simulink model "ZT_VehCtrl_18B"  (R2018b)
settings: Solver=FixedStepAuto  StartTime=0.0  StopTime=inf  FixedStep=0.005  RelTol=1e-3
InitFcn:
  | mbd_mpc_consistency_checks(bdroot(gcs));
undefined symbols (not defined in the file or in its folder): ANG_DEAD, BMS_NormalPwr, BrkPrsByBrkPct_TB_X, BrkPrsByBrkPct_TB_Y, DELAY_DISCHARGE, DELAY_RCUOFF, DRV_BACKWARD, DRV_BRAKE, DRV_FORWARD, DRV_NEUTRAL, DRV_PARK, DRV_UNPARK, DRV_ZEROTURN, EPB_LOCK, EPB_UNLOCK, ExtraLoadPwr, FanOff, fifo_0_vect, fifo_1_vect, HiFanReq, HV_finished, HV_No_Active, HV_POWER_OFF, HV_POWER_ON, HVDown, HVON, KaTLS_v_DrgUp_X_VehSpd, KeFTM_s_Way1OffDlyTime, KeFTM_TK_Way1CoolLv2OffBatTemp, KeFTM_TK_Way1CoolLv2OffMtrTemp, KeFTM_TK_Way1CoolLv2OnBatTemp, KeFTM_TK_Way1CoolLv2OnMtrTemp, KeFTM_TK_Way1CoolLv3OffBatTemp, KeFTM_TK_Way1CoolLv3OffMtrTemp, KeFTM_TK_Way1CoolLv3OnBatTemp, KeFTM_TK_Way1CoolLv3OnMtrTemp, KeFTM_TK_Way1CoolLv4OffBatTemp, KeFTM_TK_Way1CoolLv4OffMtrTemp, KeFTM_TK_Way1CoolLv4OnBatTemp, KeFTM_TK_Way1CoolLv4OnMtrTemp, Kp1, Kp2, LowFanReq, LQFP, MtrPwrFactor_RCU, MtrPwrHighToMidThd, MtrPwrLowToMidThd, MtrPwrMidToHighThd, MtrPwrMidToLowThd, MtrTrqMax, PCT_DEAD, Precharge, PTO_1000, PTO_540, pts1_fifo_0_vect, pts1_fifo_1_vect, pts2_fifo_0_vect, pts2_fifo_1_vect, pts3_fifo_0_vect, pts3_fifo_1_vect ... (+24)
libraries: mbd_mpc574x_ec_toolbox x173, canmsglib x72, simulink x57
(part 3 of 12)

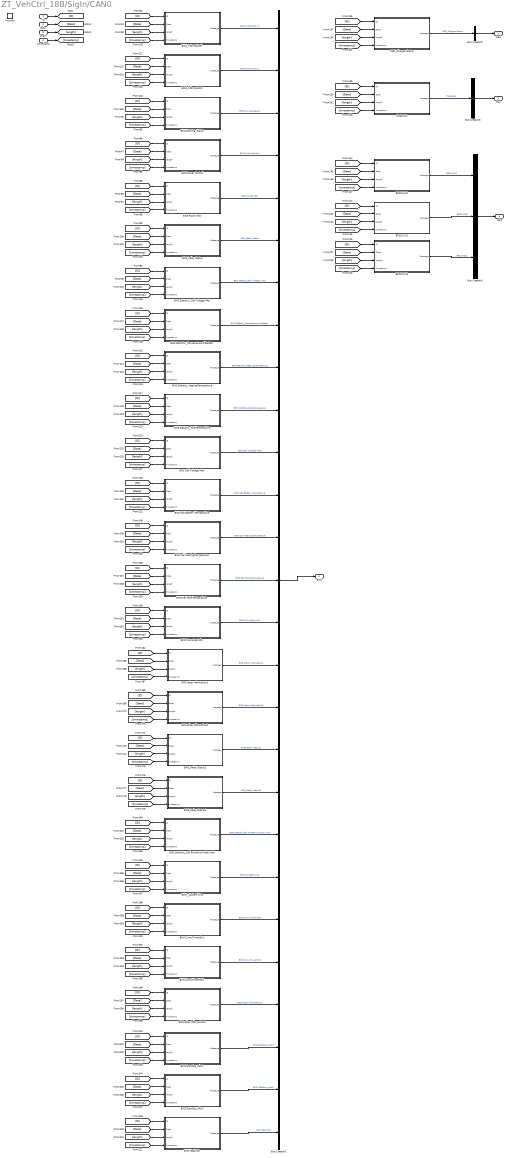
== system ZT_VehCtrl_18B/SigIn/CAN0  ==
  ID : Inport
  Data : Inport  Port=2
  length : Inport  Port=3
  timestamp : Inport  Port=4
  function : TriggerPort  TriggerType=function-call  VariantControl=Variant
  BMS Cell Battery Temperature : Subsystem
  BMS Cell HeatingTemperature : Subsystem
  BMS Cell Pole Temperature : Subsystem
  BMS Cell Voltage Infor : Subsystem
  BMS CumuCap Infor : Subsystem
  BMS CumuTimeInfor1 : Subsystem
  BMS CumuTimeInfor2 : Subsystem
  BMS HeatInfor : Subsystem
  BMS Power Control : Subsystem
  BMS Power Infor : Subsystem
  BMS StartDia_Infor1 : Subsystem
  BMS StartDia_Infor2 : Subsystem
  BMS Statistic_Cell ExtremumIndex Infor : Subsystem
  BMS Statistic_Cell Voltage Infor : Subsystem
  BMS Statistic_HeatingTemperature : Subsystem
  BMS Statistic_PoleTemperature : Subsystem
  BMS Statistic_Temperature of Battery : Subsystem
  "BMS _SystemTime " : Subsystem
  BMS other Information1 : Subsystem
  "BMS other Information2 " : Subsystem
  BMS other Information3 : Subsystem
  BMSWarning_Status : Subsystem
  BMS_Information1 : Subsystem
  BMS_Information2 : Subsystem
  BMS_Relay Status : Subsystem
  BMS_Relay Status2 : Subsystem
  BMS_Relay Status3 : Subsystem
  BRS2VCU1 : Subsystem
  BRS2VCU2 : Subsystem
  BRS2VCU3 : Subsystem
  Bus Creator5 : BusCreator  Inputs=27
  Bus Creator6 : BusCreator  Inputs=1
  Bus Creator8 : BusCreator  Inputs=1
  Bus Creator9 : BusCreator  Inputs=3
  OBC_Charger Status : Subsystem
  TMS2VCU : Subsystem
  BMS : Outport
  OBC : Outport  Port=2
  TMS : Outport  Port=3
  "BRS " : Outport  Port=4
  wires:
  [timestamp] -> BMS Statistic_Temperature of Battery/4(timestamp)
  [ID] -> BMS Cell Battery Temperature/1(ID)
  BMS Statistic_PoleTemperature/1(Message) -> Bus Creator5/10  "BMS Statistic_PoleTemperature"
  [Data] -> BMS_Relay Status/2(Data)
  BMS Statistic_Temperature of Battery/1(Message) -> Bus Creator5/8  "BMS Statistic_Temperature of Battery"
  BMS Statistic_HeatingTemperature/1(Message) -> Bus Creator5/9  "BMS Statistic_HeatingTemperature"
  [length] -> BMS Cell Battery Temperature/3(length)
  [timestamp] -> BMS Statistic_Cell Voltage Infor/4(timestamp)
  [length] -> BMS Statistic_Temperature of Battery/3(length)
  BMS Power Infor/1(Message) -> Bus Creator5/5  "BMS Power Infor"
  [timestamp] -> BMS Cell Battery Temperature/4(timestamp)
  [ID] -> BMS Statistic_PoleTemperature/1(ID)
  BMS Cell Battery Temperature/1(Message) -> Bus Creator5/12  "BMS Cell Battery Temperature"
  [Data] -> BMS Statistic_Cell Voltage Infor/2(Data)
  [length] -> BMS Statistic_PoleTemperature/3(length)
  [timestamp] -> BMS Statistic_PoleTemperature/4(timestamp)
  [Data] -> BMS Power Control/2(Data)
  [Data] -> BMS Statistic_PoleTemperature/2(Data)
  [Data] -> BMS Cell Voltage Infor/2(Data)
  BMS_Relay Status/1(Message) -> Bus Creator5/6  "BMS_Relay Status"
  [timestamp] -> BMSWarning_Status/4(timestamp)
  [ID] -> BMS Statistic_Cell Voltage Infor/1(ID)
  [Data] -> BMS Statistic_Temperature of Battery/2(Data)
  [length] -> BMSWarning_Status/3(length)
  [timestamp] -> BMS Statistic_HeatingTemperature/4(timestamp)
  Bus Creator5/1 -> BMS/1
  [timestamp] -> BMS Power Control/4(timestamp)
  [Data] -> BMS Statistic_HeatingTemperature/2(Data)
  [ID] -> BMS Power Control/1(ID)
  [Data] -> BMS Power Infor/2(Data)
  BMS Statistic_Cell Voltage Infor/1(Message) -> Bus Creator5/7  "BMS Statistic_Cell Voltage Infor"
  [ID] -> BMSWarning_Status/1(ID)
  [Data] -> BMS Cell Battery Temperature/2(Data)
  [Data] -> BMSWarning_Status/2(Data)
  [length] -> BMS Power Control/3(length)
  [ID] -> BMS Cell Voltage Infor/1(ID)
  BMSWarning_Status/1(Message) -> Bus Creator5/3  "BMSWarning_Status"
  [timestamp] -> BMS Cell Voltage Infor/4(timestamp)
  [length] -> BMS Statistic_HeatingTemperature/3(length)
  [timestamp] -> BMS_Relay Status/4(timestamp)
  [ID] -> BMS Statistic_HeatingTemperature/1(ID)
  [length] -> BMS Statistic_Cell Voltage Infor/3(length)
  [length] -> BMS_Relay Status/3(length)
  BMS Power Control/1(Message) -> Bus Creator5/4  "BMS Power Control"
  [ID] -> BMS Power Infor/1(ID)
  [length] -> BMS Cell Voltage Infor/3(length)
  [timestamp] -> BMS Power Infor/4(timestamp)
  [ID] -> BMS Statistic_Temperature of Battery/1(ID)
  BMS Cell Voltage Infor/1(Message) -> Bus Creator5/11  "BMS Cell Voltage Infor"
  [ID] -> BMS_Relay Status/1(ID)
  [length] -> BMS Power Infor/3(length)
  [Data] -> OBC_Charger Status/2(Data)
  OBC_Charger Status/1(Message) -> Bus Creator6/1  "OBC_Charger Status"
  [length] -> OBC_Charger Status/3(length)
  [ID] -> OBC_Charger Status/1(ID)
  Bus Creator6/1 -> OBC/1
  [timestamp] -> OBC_Charger Status/4(timestamp)
  BMS_Information2/1(Message) -> Bus Creator5/2  "BMS_Information2"
  BMS_Information1/1(Message) -> Bus Creator5/1  "BMS_Information1"
  [ID] -> BMS_Information2/1(ID)
  [Data] -> BMS_Information2/2(Data)
  [length] -> BMS_Information2/3(length)
  [timestamp] -> BMS_Information1/4(timestamp)
  [length] -> BMS_Information1/3(length)
  [Data] -> BMS_Information1/2(Data)
  [ID] -> BMS_Information1/1(ID)
  [timestamp] -> BMS_Information2/4(timestamp)
  [Data] -> BMS Cell HeatingTemperature/2(Data)
  BMS Cell HeatingTemperature/1(Message) -> Bus Creator5/13  "BMS Cell HeatingTemperature"
  [timestamp] -> BMS Cell HeatingTemperature/4(timestamp)
  [length] -> BMS Cell HeatingTemperature/3(length)
  [ID] -> BMS Cell HeatingTemperature/1(ID)
  [ID] -> BMS Cell Pole Temperature/1(ID)
  [length] -> BMS Cell Pole Temperature/3(length)
  [timestamp] -> BMS Cell Pole Temperature/4(timestamp)
  BMS Cell Pole Temperature/1(Message) -> Bus Creator5/14  "BMS Cell Pole Temperature"
  [Data] -> BMS Cell Pole Temperature/2(Data)
  [Data] -> BMS CumuCap Infor/2(Data)
  BMS CumuCap Infor/1(Message) -> Bus Creator5/15  "BMS CumuCap Infor"
  [timestamp] -> BMS CumuCap Infor/4(timestamp)
  [length] -> BMS CumuCap Infor/3(length)
  [ID] -> BMS CumuCap Infor/1(ID)
  [ID] -> BMS other Information1/1(ID)
  [length] -> BMS other Information1/3(length)
  [timestamp] -> BMS other Information1/4(timestamp)
  BMS other Information1/1(Message) -> Bus Creator5/16  "BMS other Information1"
  [Data] -> BMS other Information1/2(Data)
  [Data] -> "BMS other Information2 "/2(Data)
  "BMS other Information2 "/1(Message) -> Bus Creator5/17  "BMS other Information2"
  [timestamp] -> "BMS other Information2 "/4(timestamp)
  [length] -> "BMS other Information2 "/3(length)
  [ID] -> "BMS other Information2 "/1(ID)
  [ID] -> BMS_Relay Status2/1(ID)
  [length] -> BMS_Relay Status2/3(length)
  [timestamp] -> BMS_Relay Status2/4(timestamp)
  BMS_Relay Status2/1(Message) -> Bus Creator5/18  "BMS_Relay Status2"
  [Data] -> BMS_Relay Status2/2(Data)
  [Data] -> BMS_Relay Status3/2(Data)
  BMS_Relay Status3/1(Message) -> Bus Creator5/19  "BMS_Relay Status3"
  [timestamp] -> BMS_Relay Status3/4(timestamp)
  [length] -> BMS_Relay Status3/3(length)
  [ID] -> BMS_Relay Status3/1(ID)
  [ID] -> BMS Statistic_Cell ExtremumIndex Infor/1(ID)
  [length] -> BMS Statistic_Cell ExtremumIndex Infor/3(length)
  [timestamp] -> BMS Statistic_Cell ExtremumIndex Infor/4(timestamp)
  BMS Statistic_Cell ExtremumIndex Infor/1(Message) -> Bus Creator5/20  "BMS Statistic_Cell ExtremumIndex Infor"
  [Data] -> BMS Statistic_Cell ExtremumIndex Infor/2(Data)
  [Data] -> "BMS _SystemTime "/2(Data)
  "BMS _SystemTime "/1(Message) -> Bus Creator5/21  "BMS _SystemTime"
  [timestamp] -> "BMS _SystemTime "/4(timestamp)
  [length] -> "BMS _SystemTime "/3(length)
  [ID] -> "BMS _SystemTime "/1(ID)
  [ID] -> BMS CumuTimeInfor1/1(ID)
  [length] -> BMS CumuTimeInfor1/3(length)
  [timestamp] -> BMS CumuTimeInfor1/4(timestamp)
  BMS CumuTimeInfor1/1(Message) -> Bus Creator5/22  "BMS CumuTimeInfor1"
  [Data] -> BMS CumuTimeInfor1/2(Data)
  [Data] -> BMS CumuTimeInfor2/2(Data)
  BMS CumuTimeInfor2/1(Message) -> Bus Creator5/23  "BMS CumuTimeInfor2"
  [timestamp] -> BMS CumuTimeInfor2/4(timestamp)
  [length] -> BMS CumuTimeInfor2/3(length)
  [ID] -> BMS CumuTimeInfor2/1(ID)
  [ID] -> BMS other Information3/1(ID)
  [length] -> BMS other Information3/3(length)
  [timestamp] -> BMS other Information3/4(timestamp)
  BMS other Information3/1(Message) -> Bus Creator5/24  "BMS other Information3"
  [Data] -> BMS other Information3/2(Data)
  [Data] -> BMS StartDia_Infor1/2(Data)
  BMS StartDia_Infor1/1(Message) -> Bus Creator5/25  "BMS StartDia_Infor1"
  [timestamp] -> BMS StartDia_Infor1/4(timestamp)
  [length] -> BMS StartDia_Infor1/3(length)
  [ID] -> BMS StartDia_Infor1/1(ID)
  [ID] -> BMS StartDia_Infor2/1(ID)
  [length] -> BMS StartDia_Infor2/3(length)
  [timestamp] -> BMS StartDia_Infor2/4(timestamp)
  BMS StartDia_Infor2/1(Message) -> Bus Creator5/26  "BMS StartDia_Infor2"
  [Data] -> BMS StartDia_Infor2/2(Data)
  [Data] -> BMS HeatInfor/2(Data)
  BMS HeatInfor/1(Message) -> Bus Creator5/27  "BMS HeatInfor"
  [timestamp] -> BMS HeatInfor/4(timestamp)
  [length] -> BMS HeatInfor/3(length)
  [ID] -> BMS HeatInfor/1(ID)
  [timestamp] -> TMS2VCU/4(timestamp)
  Bus Creator8/1 -> TMS/1
  [ID] -> TMS2VCU/1(ID)
  [length] -> TMS2VCU/3(length)
  TMS2VCU/1(Message) -> Bus Creator8/1  "TMS2VCU"
  [Data] -> TMS2VCU/2(Data)
  [Data] -> BRS2VCU1/2(Data)
  BRS2VCU1/1(Message) -> Bus Creator9/1  "BRS2VCU1"
  [length] -> BRS2VCU1/3(length)
  [ID] -> BRS2VCU1/1(ID)
  Bus Creator9/1 -> "BRS "/1
  [timestamp] -> BRS2VCU1/4(timestamp)
  [timestamp] -> BRS2VCU2/4(timestamp)
  [ID] -> BRS2VCU2/1(ID)
  [length] -> BRS2VCU2/3(length)
  [Data] -> BRS2VCU2/2(Data)
  [Data] -> BRS2VCU3/2(Data)
  [length] -> BRS2VCU3/3(length)
  [ID] -> BRS2VCU3/1(ID)
  [timestamp] -> BRS2VCU3/4(timestamp)
  BRS2VCU2/1(Message) -> Bus Creator9/2  "BRS2VCU2"
  BRS2VCU3/1(Message) -> Bus Creator9/3  "BRS2VCU3"
  length/1 -> [length]
  ID/1 -> [ID]
  timestamp/1 -> [timestamp]
  Data/1 -> [Data]

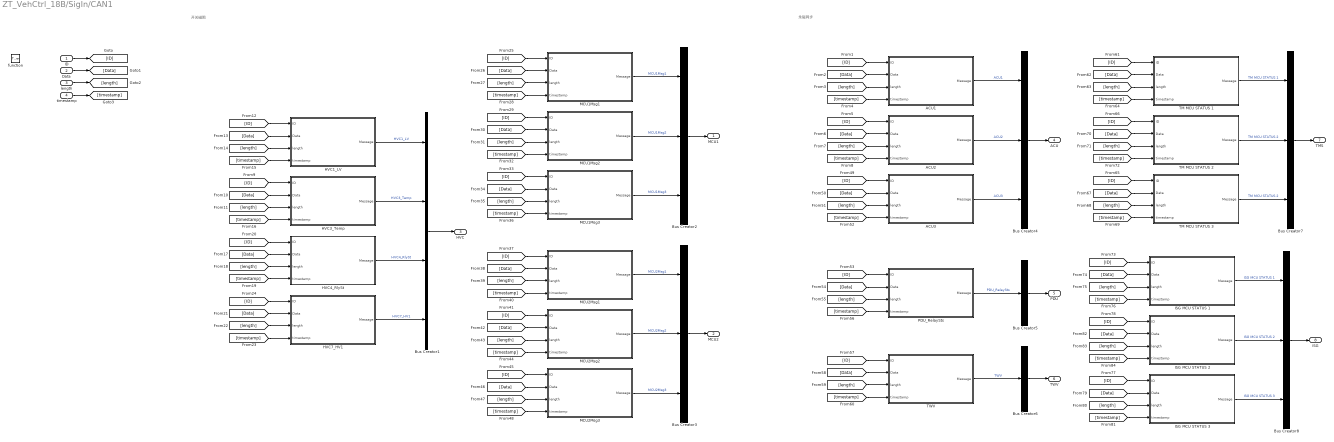
== system ZT_VehCtrl_18B/SigIn/CAN1 ==
  note: 永磁同步
  note: 开关磁阻
  ID : Inport
  Data : Inport  Port=2
  length : Inport  Port=3
  timestamp : Inport  Port=4
  function : TriggerPort  TriggerType=function-call  VariantControl=Variant
  ACU1 : Subsystem
  ACU2 : Subsystem
  ACU3 : Subsystem
  Bus Creator1 : BusCreator  Inputs=4
  Bus Creator{2..4,7..8} (5 alike) : BusCreator  Inputs=3
  Bus Creator5 : BusCreator  Inputs=1
  Bus Creator6 : BusCreator  Inputs=1
  HVC1_LV : Subsystem
  HVC3_Temp : Subsystem
  HVC4_RlySt : Subsystem
  HVC7_HV1 : Subsystem
  ISG MCU STATUS 1 : Subsystem
  ISG MCU STATUS 2 : Subsystem
  ISG MCU STATUS 3 : Subsystem
  MCU1Msg1 : Subsystem
  MCU1Msg2 : Subsystem
  MCU1Msg3 : Subsystem
  MCU2Msg1 : Subsystem
  MCU2Msg2 : Subsystem
  MCU2Msg3 : Subsystem
  PDU_RelaySts : Subsystem
  TM MCU STATUS 1 : Subsystem
  TM MCU STATUS 2 : Subsystem
  TM MCU STATUS 3 : Subsystem
  "TWV " : Subsystem
  MCU1 : Outport
  MCU2 : Outport  Port=2
  HVC : Outport  Port=3
  ACU : Outport  Port=4
  PDU : Outport  Port=5
  TWV : Outport  Port=6
  TMS : Outport  Port=7
  "ISG " : Outport  Port=8
  wires:
  length/1 -> [length]
  timestamp/1 -> [timestamp]
  Data/1 -> [Data]
  ID/1 -> [ID]
  Bus Creator2/1 -> MCU1/1
  [Data] -> HVC1_LV/2(Data)
  [timestamp] -> HVC1_LV/4(timestamp)
  [ID] -> HVC1_LV/1(ID)
  HVC1_LV/1(Message) -> Bus Creator1/1  "HVC1_LV"
  [length] -> HVC1_LV/3(length)
  [length] -> HVC3_Temp/3(length)
  HVC3_Temp/1(Message) -> Bus Creator1/2  "HVC3_Temp"
  [ID] -> HVC3_Temp/1(ID)
  [timestamp] -> HVC3_Temp/4(timestamp)
  [Data] -> HVC3_Temp/2(Data)
  [Data] -> HVC4_RlySt/2(Data)
  [timestamp] -> HVC4_RlySt/4(timestamp)
  [ID] -> HVC4_RlySt/1(ID)
  [length] -> HVC4_RlySt/3(length)
  HVC4_RlySt/1(Message) -> Bus Creator1/3  "HVC4_RlySt"
  HVC7_HV1/1(Message) -> Bus Creator1/4  "HVC7_HV1"
  [length] -> HVC7_HV1/3(length)
  [ID] -> HVC7_HV1/1(ID)
  [timestamp] -> HVC7_HV1/4(timestamp)
  [Data] -> HVC7_HV1/2(Data)
  [length] -> MCU1Msg1/3(length)
  MCU1Msg1/1(Message) -> Bus Creator2/1  "MCU1Msg1"
  [ID] -> MCU1Msg1/1(ID)
  [timestamp] -> MCU1Msg1/4(timestamp)
  [Data] -> MCU1Msg1/2(Data)
  [Data] -> MCU1Msg2/2(Data)
  [timestamp] -> MCU1Msg2/4(timestamp)
  [ID] -> MCU1Msg2/1(ID)
  MCU1Msg2/1(Message) -> Bus Creator2/2  "MCU1Msg2"
  [length] -> MCU1Msg2/3(length)
  [length] -> MCU1Msg3/3(length)
  [ID] -> MCU1Msg3/1(ID)
  [timestamp] -> MCU1Msg3/4(timestamp)
  [Data] -> MCU1Msg3/2(Data)
  MCU1Msg3/1(Message) -> Bus Creator2/3  "MCU1Msg3"
  MCU2Msg3/1(Message) -> Bus Creator3/3  "MCU2Msg3"
  [Data] -> MCU2Msg3/2(Data)
  [timestamp] -> MCU2Msg3/4(timestamp)
  [ID] -> MCU2Msg3/1(ID)
  [length] -> MCU2Msg3/3(length)
  [length] -> MCU2Msg2/3(length)
  MCU2Msg2/1(Message) -> Bus Creator3/2  "MCU2Msg2"
  [ID] -> MCU2Msg2/1(ID)
  [timestamp] -> MCU2Msg2/4(timestamp)
  [Data] -> MCU2Msg2/2(Data)
  [Data] -> MCU2Msg1/2(Data)
  [timestamp] -> MCU2Msg1/4(timestamp)
  [ID] -> MCU2Msg1/1(ID)
  MCU2Msg1/1(Message) -> Bus Creator3/1  "MCU2Msg1"
  [length] -> MCU2Msg1/3(length)
  ACU3/1(Message) -> Bus Creator4/3  "ACU3"
  [Data] -> ACU3/2(Data)
  [timestamp] -> ACU3/4(timestamp)
  [ID] -> ACU3/1(ID)
  [length] -> ACU3/3(length)
  [length] -> ACU2/3(length)
  ACU2/1(Message) -> Bus Creator4/2  "ACU2"
  [ID] -> ACU2/1(ID)
  [timestamp] -> ACU2/4(timestamp)
  [Data] -> ACU2/2(Data)
  [Data] -> ACU1/2(Data)
  [timestamp] -> ACU1/4(timestamp)
  [ID] -> ACU1/1(ID)
  ACU1/1(Message) -> Bus Creator4/1  "ACU1"
  [length] -> ACU1/3(length)
  Bus Creator4/1 -> ACU/1
  [length] -> PDU_RelaySts/3(length)
  [ID] -> PDU_RelaySts/1(ID)
  [timestamp] -> PDU_RelaySts/4(timestamp)
  [Data] -> PDU_RelaySts/2(Data)
  PDU_RelaySts/1(Message) -> Bus Creator5/1  "PDU_RelaySts"
  Bus Creator5/1 -> PDU/1
  Bus Creator6/1 -> TWV/1
  "TWV "/1(Message) -> Bus Creator6/1  "TWV"
  [Data] -> "TWV "/2(Data)
  [timestamp] -> "TWV "/4(timestamp)
  [ID] -> "TWV "/1(ID)
  [length] -> "TWV "/3(length)
  Bus Creator7/1 -> TMS/1
  [length] -> TM MCU STATUS 1/3(length)
  TM MCU STATUS 1/1(Message) -> Bus Creator7/1  "TM MCU STATUS 1"
  [ID] -> TM MCU STATUS 1/1(ID)
  [timestamp] -> TM MCU STATUS 1/4(timestamp)
  [Data] -> TM MCU STATUS 1/2(Data)
  [Data] -> TM MCU STATUS 2/2(Data)
  [timestamp] -> TM MCU STATUS 2/4(timestamp)
  [ID] -> TM MCU STATUS 2/1(ID)
  TM MCU STATUS 2/1(Message) -> Bus Creator7/2  "TM MCU STATUS 2"
  [length] -> TM MCU STATUS 2/3(length)
  [length] -> TM MCU STATUS 3/3(length)
  [ID] -> TM MCU STATUS 3/1(ID)
  [timestamp] -> TM MCU STATUS 3/4(timestamp)
  [Data] -> TM MCU STATUS 3/2(Data)
  TM MCU STATUS 3/1(Message) -> Bus Creator7/3  "TM MCU STATUS 2"
  ISG MCU STATUS 3/1(Message) -> Bus Creator8/3  "ISG MCU STATUS 3"
  [Data] -> ISG MCU STATUS 3/2(Data)
  [timestamp] -> ISG MCU STATUS 3/4(timestamp)
  [ID] -> ISG MCU STATUS 3/1(ID)
  [length] -> ISG MCU STATUS 3/3(length)
  [length] -> ISG MCU STATUS 2/3(length)
  ISG MCU STATUS 2/1(Message) -> Bus Creator8/2  "ISG MCU STATUS 2"
  [ID] -> ISG MCU STATUS 2/1(ID)
  [timestamp] -> ISG MCU STATUS 2/4(timestamp)
  [Data] -> ISG MCU STATUS 2/2(Data)
  [Data] -> ISG MCU STATUS 1/2(Data)
  [timestamp] -> ISG MCU STATUS 1/4(timestamp)
  [ID] -> ISG MCU STATUS 1/1(ID)
  ISG MCU STATUS 1/1(Message) -> Bus Creator8/1  "ISG MCU STATUS 1"
  [length] -> ISG MCU STATUS 1/3(length)
  Bus Creator8/1 -> "ISG "/1
  Bus Creator1/1 -> HVC/1
  Bus Creator3/1 -> MCU2/1

== system ZT_VehCtrl_18B/SigIn/DI ==
  note: DI PULLDOWN
  note: DI PULLUP
  Bus Creator : BusCreator  Inputs=14
  DI01 : mbd_mpc574x_ec_toolbox/GPIO Blocks/Digital_Input  gpio_pin=PTG5: [SIUL2_GPIO101 | General Purpose IO PG[5]]  pull_resistor=None
  DI02 : mbd_mpc574x_ec_toolbox/GPIO Blocks/Digital_Input  gpio_pin=PTG9: [SIUL2_GPIO105 | General Purpose IO PG[9]]  pull_resistor=None
  DI03 : mbd_mpc574x_ec_toolbox/GPIO Blocks/Digital_Input  gpio_pin=PTC11: [SIUL2_GPIO43 | General Purpose IO PC[11]]  pull_resistor=None
  DI04 : mbd_mpc574x_ec_toolbox/GPIO Blocks/Digital_Input  gpio_pin=PTA9: [SIUL2_GPIO9 | General Purpose IO PA[9]]  pull_resistor=None
  DI07 : mbd_mpc574x_ec_toolbox/GPIO Blocks/Digital_Input  gpio_pin=PTA0: [SIUL2_GPIO0 | General Purpose IO PA[0]]  pull_resistor=None
  DI08 : mbd_mpc574x_ec_toolbox/GPIO Blocks/Digital_Input  gpio_pin=PTD11: [SIUL2_GPIO59 | General Purpose IO PD[11]]  pull_resistor=None
  DI09 : mbd_mpc574x_ec_toolbox/GPIO Blocks/Digital_Input  gpio_pin=PTG6: [SIUL2_GPIO102 | General Purpose IO PG[6]]  pull_resistor=None
  DI10 : mbd_mpc574x_ec_toolbox/GPIO Blocks/Digital_Input  gpio_pin=PTG2: [SIUL2_GPIO98 | General Purpose IO PG[2]]  pull_resistor=None
  DI12 : mbd_mpc574x_ec_toolbox/GPIO Blocks/Digital_Input  gpio_pin=PTF13: [SIUL2_GPIO93 | General Purpose IO PF[13]]  pull_resistor=None
  DI13 : mbd_mpc574x_ec_toolbox/GPIO Blocks/Digital_Input  gpio_pin=PTG4: [SIUL2_GPIO100 | General Purpose IO PG[4]]  pull_resistor=None
  DI15 : mbd_mpc574x_ec_toolbox/GPIO Blocks/Digital_Input  gpio_pin=PTF12: [SIUL2_GPIO92 | General Purpose IO PF[12]]  pull_resistor=None
  DI16 : mbd_mpc574x_ec_toolbox/GPIO Blocks/Digital_Input  gpio_pin=PTG7: [SIUL2_GPIO103 | General Purpose IO PG[7]]  pull_resistor=None
  DI17 : mbd_mpc574x_ec_toolbox/GPIO Blocks/Digital_Input  gpio_pin=PTD10: [SIUL2_GPIO58 | General Purpose IO PD[10]]  pull_resistor=None
  DI18 : mbd_mpc574x_ec_toolbox/GPIO Blocks/Digital_Input  gpio_pin=PTG10: [SIUL2_GPIO106 | General Purpose IO PG[10]]  pull_resistor=None
  DI_31_32_33_34 : Subsystem  Commented=on
  Data Store Read : DataStoreRead  DataStoreName=DI07
  Data Store Read1 : DataStoreRead  DataStoreName=DI10
  Data Store Read10 : DataStoreRead  DataStoreName=DI04
  Data Store Read11 : DataStoreRead  DataStoreName=DI12
  Data Store Read12 : DataStoreRead  DataStoreName=DI08
  Data Store Read13 : DataStoreRead  DataStoreName=DI09
  Data Store Read2 : DataStoreRead  DataStoreName=DI13
  Data Store Read3 : DataStoreRead  DataStoreName=DI15
  Data Store Read4 : DataStoreRead  DataStoreName=DI16
  Data Store Read5 : DataStoreRead  DataStoreName=DI17
  Data Store Read6 : DataStoreRead  DataStoreName=DI18
  Data Store Read7 : DataStoreRead  DataStoreName=DI01
  Data Store Read8 : DataStoreRead  DataStoreName=DI02
  Data Store Read9 : DataStoreRead  DataStoreName=DI03
  Data Store Write : DataStoreWrite  DataStoreName=DI07
  Data Store Write1 : DataStoreWrite  DataStoreName=DI01
  Data Store Write10 : DataStoreWrite  DataStoreName=DI04
  Data Store Write11 : DataStoreWrite  DataStoreName=DI12
  Data Store Write12 : DataStoreWrite  DataStoreName=DI08
  Data Store Write13 : DataStoreWrite  DataStoreName=DI09
  Data Store Write2 : DataStoreWrite  DataStoreName=DI10
  Data Store Write3 : DataStoreWrite  DataStoreName=DI13
  Data Store Write4 : DataStoreWrite  DataStoreName=DI15
  Data Store Write5 : DataStoreWrite  DataStoreName=DI16
  Data Store Write6 : DataStoreWrite  DataStoreName=DI17
  Data Store Write7 : DataStoreWrite  DataStoreName=DI18
  Data Store Write8 : DataStoreWrite  DataStoreName=DI02
  Data Store Write9 : DataStoreWrite  DataStoreName=DI03
  DI : Outport
  wires:
  DI07/1 -> Data Store Write/1
  DI01/1 -> Data Store Write1/1
  DI10/1 -> Data Store Write2/1
  DI13/1 -> Data Store Write3/1
  DI15/1 -> Data Store Write4/1
  DI17/1 -> Data Store Write6/1
  DI16/1 -> Data Store Write5/1
  DI18/1 -> Data Store Write7/1
  DI09/1 -> Data Store Write13/1
  DI08/1 -> Data Store Write12/1
  DI12/1 -> Data Store Write11/1
  DI04/1 -> Data Store Write10/1
  DI02/1 -> Data Store Write8/1
  DI03/1 -> Data Store Write9/1
  Data Store Read/1 -> Bus Creator/1  "DI07"
  Data Store Read1/1 -> Bus Creator/2  "DI10"
  Data Store Read2/1 -> Bus Creator/3  "DI13"
  Data Store Read3/1 -> Bus Creator/4  "DI15"
  Data Store Read4/1 -> Bus Creator/5  "DI16"
  Data Store Read5/1 -> Bus Creator/6  "DI17"
  Data Store Read6/1 -> Bus Creator/7  "DI18"
  Data Store Read7/1 -> Bus Creator/8  "DI01"
  Data Store Read8/1 -> Bus Creator/9  "DI02"
  Data Store Read9/1 -> Bus Creator/10  "DI03"
  Data Store Read10/1 -> Bus Creator/11  "DI04"
  Data Store Read11/1 -> Bus Creator/12  "DI12"
  Data Store Read12/1 -> Bus Creator/13  "DI08"
  Data Store Read13/1 -> Bus Creator/14  "DI09"
  Bus Creator/1 -> DI/1

== system ZT_VehCtrl_18B/SigIn/PWM ==
  note: DI PWM PULLDOWN
  note: DI PWM PULLUP
  Bus Creator : BusCreator  Inputs=8
  Data Store Read : DataStoreRead  DataStoreName=DI31_PWM_DC
  Data Store Read1 : DataStoreRead  DataStoreName=DI31_PWM_FRQ
  Data Store Read2 : DataStoreRead  DataStoreName=DI32_PWM_DC
  Data Store Read3 : DataStoreRead  DataStoreName=DI32_PWM_FRQ
  Data Store Read4 : DataStoreRead  DataStoreName=DI33_PWM_DC
  Data Store Read5 : DataStoreRead  DataStoreName=DI33_PWM_FRQ
  Data Store Read6 : DataStoreRead  DataStoreName=DI34_PWM_DC
  Data Store Read7 : DataStoreRead  DataStoreName=DI34_PWM_FRQ
  Data Store Write : DataStoreWrite  DataStoreName=DI31_PWM_DC
  Data Store Write1 : DataStoreWrite  DataStoreName=DI31_PWM_FRQ
  Data Store Write2 : DataStoreWrite  DataStoreName=DI32_PWM_DC
  Data Store Write3 : DataStoreWrite  DataStoreName=DI32_PWM_FRQ
  Data Store Write4 : DataStoreWrite  DataStoreName=DI33_PWM_DC
  Data Store Write5 : DataStoreWrite  DataStoreName=DI33_PWM_FRQ
  Data Store Write6 : DataStoreWrite  DataStoreName=DI34_PWM_FRQ
  Data Store Write7 : DataStoreWrite  DataStoreName=DI34_PWM_DC
  PWM_PTS1 : Subsystem
  PWM_PTS2 : Subsystem
  PWM_PTS3 : Subsystem
  PWM_PTS4 : Subsystem
  Subsystem : Subsystem  Commented=on
  eTimer_Arm_Capture : mbd_mpc574x_ec_toolbox/Motor Control Blocks/eTIMER Blocks/eTimer_Arm_Capture  etimerModule=0  etimerChannel=2  etimerArmAction=Start
  eTimer_Arm_Capture1 : mbd_mpc574x_ec_toolbox/Motor Control Blocks/eTIMER Blocks/eTimer_Arm_Capture  etimerModule=1  etimerChannel=2  etimerArmAction=Start
  eTimer_Arm_Capture2 : mbd_mpc574x_ec_toolbox/Motor Control Blocks/eTIMER Blocks/eTimer_Arm_Capture  etimerModule=1  etimerChannel=1  etimerArmAction=Start
  eTimer_Arm_Capture3 : mbd_mpc574x_ec_toolbox/Motor Control Blocks/eTIMER Blocks/eTimer_Arm_Capture  etimerModule=1  etimerChannel=3  etimerArmAction=Start
  PWMIn : Outport
  wires:
  Bus Creator/1 -> PWMIn/1
  Data Store Read7/1 -> Bus Creator/8  "DI34_PWM_FRQ"
  Data Store Read6/1 -> Bus Creator/7  "DI34_PWM_DC"
  Data Store Read5/1 -> Bus Creator/6  "DI33_PWM_FRQ"
  Data Store Read4/1 -> Bus Creator/5  "DI33_PWM_DC"
  Data Store Read3/1 -> Bus Creator/4  "DI32_PWM_FRQ"
  Data Store Read2/1 -> Bus Creator/3  "DI32_PWM_DC"
  Data Store Read1/1 -> Bus Creator/2  "DI31_PWM_FRQ"
  Data Store Read/1 -> Bus Creator/1  "DI31_PWM_DC"
  PWM_PTS4/1(DC) -> Data Store Write/1
  PWM_PTS4/2(freq) -> Data Store Write1/1
  PWM_PTS1/1(DC) -> Data Store Write2/1
  PWM_PTS1/2(freq) -> Data Store Write3/1
  PWM_PTS2/1(DC) -> Data Store Write4/1
  PWM_PTS2/2(freq) -> Data Store Write5/1
  PWM_PTS3/2(freq) -> Data Store Write6/1
  PWM_PTS3/1(DC) -> Data Store Write7/1

== system ZT_VehCtrl_18B/SigOut/ACU ==
  "ACU_OUT " : Inport
  Trigger : TriggerPort  VariantControl=Variant  PortDimensions=1
  Bus Selector : BusSelector  OutputSignals=Data,Length
  FCAN_Send_ID_0x0C079AA7 : mbd_mpc574x_ec_toolbox/Communication Blocks/CAN Blocks/FCAN_Send  Priority=2  can_instance=1  can_mode=Non-blocking  can_timeout_ms=0  can_mb_idx=43  can_extended_id=on  can_is_remote=off  can_id=0C079AA7  show_adv_opts=off  can_fd_enable=off  can_enable_brs=off  can_fd_padding=0
      settings: SourceProductName=NXP Model-Based Design Toolbox for MPC57xx MCUs
  VCU_ACU1 : canmsglib/CAN Pack  CANdbFile=D:\VCU\VCU_SL_ZhengZhou\ZT2\模型与接口\CAN_DBC\动力CANB_GBK.dbc  MsgList=VCU_ACU1  MsgName=VCU_ACU1  MsgIDType=Extended (29-bit identifier)  MsgIdentifier=201824935  MsgLength=8  SignalInfo=DcacAcCmd$32$8$1$2$1$0$1$0$-Inf$Inf$#DcacEpsCmd$16$8$1$2$1$0$1$0$-Inf$Inf$#DcacEpsMode$24$8$1$2$1$0$1$0$-Inf$Inf$#DcdcCmd$0$8$1$2$1$0$1$0$-Inf$Inf$#  NSignals=4  StartBits=str2num('[int32(32);int32(16);int32(24);int32(0)]')  SignalSizes=str2num('[int32(8);int32(8);int32(8);int32(8)]')  ByteOrders=str2num('[int32(1);int32(1);int32(1);int32(1)]')  DataTypes=str2num('[int32(2);int32(2);int32(2);int32(2)]')  MultiplexTypes=str2num('[int32(1);int32(1);int32(1);int32(1)]')  MultiplexValues=str2num('[double(0);double(0);double(0);double(0)]')  Factors=str2num('[double(1);double(1);double(1);double(1)]')  Offsets=str2num('[double(0);double(0);double(0);double(0)]')  Minimums=str2num('[double(-Inf);double(-Inf);double(-Inf);double(-Inf)]')  Maximums=str2num('[double(Inf);double(Inf);double(Inf);double(Inf)]')  Remote=off  ApplyMinMax=off  BusOutput=on
      settings: SourceProductName=Simulink Real-Time  SourceProductBaseCode=XP  DataFormat=CANdb specified signals
  wires:
  VCU_ACU1/1 -> Bus Selector/1
  Bus Selector/2 -> FCAN_Send_ID_0x0C079AA7/2  "<Length>"
  Bus Selector/1 -> FCAN_Send_ID_0x0C079AA7/1  "<Data>"

== system ZT_VehCtrl_18B/SigOut/BMS ==
  "BMS_OUT " : Inport
  Trigger : TriggerPort  VariantControl=Variant  PortDimensions=1
  Bus Selector : BusSelector  OutputSignals=Data,Length
  FCAN_Send_ID_0x160 : mbd_mpc574x_ec_toolbox/Communication Blocks/CAN Blocks/FCAN_Send  Priority=2  can_instance=0  can_mode=Non-blocking  can_timeout_ms=0  can_mb_idx=43  can_extended_id=off  can_is_remote=off  can_id=160  show_adv_opts=off  can_fd_enable=off  can_enable_brs=off  can_fd_padding=0
      settings: SourceProductName=NXP Model-Based Design Toolbox for MPC57xx MCUs
  VCU_BMS : canmsglib/CAN Pack  CANdbFile=D:\VCU\VCU_SL_ZhengZhou\ZT2\模型与接口\CAN_DBC\整车CANA_GBK.dbc  MsgList=VCU_BMS  MsgName=VCU_BMS  MsgIDType=Standard (11-bit identifier)  MsgIdentifier=352  MsgLength=8  SignalInfo=VCU_PowerOnReq$0$1$2$2$1$0$1$0$0$1$#VCU_UrgencyCutOffPowerReq$1$1$2$2$1$0$1$0$0$1$#  NSignals=2  StartBits=str2num('[int32(0);int32(1)]')  SignalSizes=str2num('[int32(1);int32(1)]')  ByteOrders=str2num('[int32(2);int32(2)]')  DataTypes=str2num('[int32(2);int32(2)]')  MultiplexTypes=str2num('[int32(1);int32(1)]')  MultiplexValues=str2num('[double(0);double(0)]')  Factors=str2num('[double(1);double(1)]')  Offsets=str2num('[double(0);double(0)]')  Minimums=str2num('[double(0);double(0)]')  Maximums=str2num('[double(1);double(1)]')  Remote=off  ApplyMinMax=off  BusOutput=on
      settings: SourceProductName=Simulink Real-Time  SourceProductBaseCode=XP  DataFormat=CANdb specified signals
  wires:
  VCU_BMS/1 -> Bus Selector/1
  Bus Selector/2 -> FCAN_Send_ID_0x160/2  "<Length>"
  Bus Selector/1 -> FCAN_Send_ID_0x160/1  "<Data>"

== system ZT_VehCtrl_18B/SigOut/BRS ==
  "BRS_OUT " : Inport
  Trigger : TriggerPort  VariantControl=Variant  PortDimensions=1
  Bus Selector : BusSelector  OutputSignals=Data,Length
  Bus Selector1 : BusSelector  OutputSignals=DCDC_Enable
  FCAN_Send_ID_0x0CF109A7 : mbd_mpc574x_ec_toolbox/Communication Blocks/CAN Blocks/FCAN_Send  Priority=2  can_instance=0  can_mode=Non-blocking  can_timeout_ms=0  can_mb_idx=44  can_extended_id=on  can_is_remote=off  can_id=0CF109A7  show_adv_opts=off  can_fd_enable=off  can_enable_brs=off  can_fd_padding=0
      settings: SourceProductName=NXP Model-Based Design Toolbox for MPC57xx MCUs
  VCU2BRS : canmsglib/CAN Pack  CANdbFile=D:\VCU\VCU_SL_ZhengZhou\ZT2\模型与接口\CAN_DBC\整车CANA_GBK.dbc  MsgList=VCU2BRS  MsgName=VCU2BRS  MsgIDType=Extended (29-bit identifier)  MsgIdentifier=217123239  MsgLength=8  SignalInfo=LiveCounter$56$8$1$2$1$0$1$0$0$255$#MaxChargePowerLimit$16$16$1$2$1$0$1$0$0$500$#OnOffCmd$46$1$1$2$1$0$1$0$0$1$#PowerReq$0$16$1$2$1$0$1$0$0$500$#  NSignals=4  StartBits=str2num('[int32(56);int32(16);int32(46);int32(0)]')  SignalSizes=str2num('[int32(8);int32(16);int32(1);int32(16)]')  ByteOrders=str2num('[int32(1);int32(1);int32(1);int32(1)]')  DataTypes=str2num('[int32(2);int32(2);int32(2);int32(2)]')  MultiplexTypes=str2num('[int32(1);int32(1);int32(1);int32(1)]')  MultiplexValues=str2num('[double(0);double(0);double(0);double(0)]')  Factors=str2num('[double(1);double(1);double(1);double(1)]')  Offsets=str2num('[double(0);double(0);double(0);double(0)]')  Minimums=str2num('[double(0);double(0);double(0);double(0)]')  Maximums=str2num('[double(255);double(500);double(1);double(500)]')  Remote=off  ApplyMinMax=off  BusOutput=on
      settings: SourceProductName=Simulink Real-Time  SourceProductBaseCode=XP  DataFormat=CANdb specified signals
  wires:
  VCU2BRS/1 -> Bus Selector/1
  "BRS_OUT "/1 -> Bus Selector1/1
  Bus Selector/1 -> FCAN_Send_ID_0x0CF109A7/1  "<Data>"
  Bus Selector/2 -> FCAN_Send_ID_0x0CF109A7/2  "<Length>"

== system ZT_VehCtrl_18B/SigOut/DCDC ==
  "DCDC_OUT " : Inport
  Trigger : TriggerPort  VariantControl=Variant  PortDimensions=1
  Bus Selector : BusSelector  OutputSignals=Data,Length
  FCAN_Send_ID_0x18008FD0 : mbd_mpc574x_ec_toolbox/Communication Blocks/CAN Blocks/FCAN_Send  Priority=2  can_instance=1  can_mode=Non-blocking  can_timeout_ms=0  can_mb_idx=43  can_extended_id=on  can_is_remote=off  can_id=18008FD0  show_adv_opts=off  can_fd_enable=off  can_enable_brs=off  can_fd_padding=0
      settings: SourceProductName=NXP Model-Based Design Toolbox for MPC57xx MCUs
  VCU_DCDC1 : canmsglib/CAN Pack  CANdbFile=D:\VCU\VCU_SL_ZhengZhou\ZT2\模型与接口\CAN_DBC\动力CANB_GBK.dbc  MsgList=VCU_DCDC1  MsgName=VCU_DCDC1  MsgIDType=Extended (29-bit identifier)  MsgIdentifier=402690000  MsgLength=8  SignalInfo=VCU_DCDC1_En$0$2$1$2$1$0$1$0$0$3$#  NSignals=1  StartBits=str2num('[int32(0)]')  SignalSizes=str2num('[int32(2)]')  ByteOrders=str2num('[int32(1)]')  DataTypes=str2num('[int32(2)]')  MultiplexTypes=str2num('[int32(1)]')  MultiplexValues=str2num('[double(0)]')  Factors=str2num('[double(1)]')  Offsets=str2num('[double(0)]')  Minimums=str2num('[double(0)]')  Maximums=str2num('[double(3)]')  Remote=off  ApplyMinMax=off  BusOutput=on
      settings: SourceProductName=Simulink Real-Time  SourceProductBaseCode=XP  DataFormat=CANdb specified signals
  wires:
  VCU_DCDC1/1 -> Bus Selector/1
  Bus Selector/2 -> FCAN_Send_ID_0x18008FD0/2  "<Length>"
  Bus Selector/1 -> FCAN_Send_ID_0x18008FD0/1  "<Data>"

== system ZT_VehCtrl_18B/SigOut/GPIO  ==
  note: LS
  note: PWM
  note: HS
  ETC : Subsystem
  HS : Subsystem
  PWM_OUT : Subsystem  Commented=on
  SPI0: LS09_14_15_16_1_2_11_4 : Subsystem
  SPI3: LS03_06_07_08_10_12_13_17_18_19 : Subsystem

== system ZT_VehCtrl_18B/SigOut/HVC ==
  "HVC_OUT " : Inport
  Trigger : TriggerPort  VariantControl=Variant  PortDimensions=1
  Bus Selector : BusSelector  OutputSignals=Data,Length
  Ctrl_HVC : canmsglib/CAN Pack  CANdbFile=D:\VCU\VCU_SL_ZhengZhou\ZT2\模型与接口\CAN_DBC\动力CANB_GBK.dbc  MsgList=Ctrl_HVC  MsgName=Ctrl_HVC  MsgIDType=Extended (29-bit identifier)  MsgIdentifier=402694405  MsgLength=8  SignalInfo=EDrv1_PowOnCmd$0$1$1$2$1$0$1$0$0$1$#EDrv2_PowOnCmd$2$1$1$2$1$0$1$0$0$1$#HvcCmd_Life$60$4$1$2$1$0$1$0$0$15$#PTC_PowOnCmd$6$1$1$2$1$0$1$0$0$1$#PaxAC_PowOnCmd$4$1$1$2$1$0$1$0$0$1$#  NSignals=5  StartBits=str2num('[int32(0);int32(2);int32(60);int32(6);int32(4)]')  SignalSizes=str2num('[int32(1);int32(1);int32(4);int32(1);int32(1)]')  ByteOrders=str2num('[int32(1);int32(1);int32(1);int32(1);int32(1)]')  DataTypes=str2num('[int32(2);int32(2);int32(2);int32(2);int32(2)]')  MultiplexTypes=str2num('[int32(1);int32(1);int32(1);int32(1);int32(1)]')  MultiplexValues=str2num('[double(0);double(0);double(0);double(0);double(0)]')  Factors=str2num('[double(1);double(1);double(1);double(1);double(1)]')  Offsets=str2num('[double(0);double(0);double(0);double(0);double(0)]')  Minimums=str2num('[double(0);double(0);double(0);double(0);double(0)]')  Maximums=str2num('[double(1);double(1);double(15);double(1);double(1)]')  Remote=off  ApplyMinMax=off  BusOutput=on
      settings: SourceProductName=Simulink Real-Time  SourceProductBaseCode=XP  DataFormat=CANdb specified signals
  FCAN_Send_ID_0x1800A105 : mbd_mpc574x_ec_toolbox/Communication Blocks/CAN Blocks/FCAN_Send  Priority=2  can_instance=1  can_mode=Non-blocking  can_timeout_ms=0  can_mb_idx=43  can_extended_id=on  can_is_remote=off  can_id=1800A105  show_adv_opts=off  can_fd_enable=off  can_enable_brs=off  can_fd_padding=0
      settings: SourceProductName=NXP Model-Based Design Toolbox for MPC57xx MCUs
  wires:
  Bus Selector/1 -> FCAN_Send_ID_0x1800A105/1  "<Data>"
  Bus Selector/2 -> FCAN_Send_ID_0x1800A105/2  "<Length>"
  Ctrl_HVC/1 -> Bus Selector/1

== system ZT_VehCtrl_18B/SigOut/ICU1  ==
  "ICU_OUT " : Inport
  Trigger : TriggerPort  VariantControl=Variant  PortDimensions=1
  Bus Selector{,3..7} (6 alike) : BusSelector  OutputSignals=Data,Length
  Bus Selector1 : BusSelector  OutputSignals=DCDC_Enable
  FCAN_Send_ID_0x180128D0 : mbd_mpc574x_ec_toolbox/Communication Blocks/CAN Blocks/FCAN_Send  Priority=2  can_instance=0  can_mode=Non-blocking  can_timeout_ms=0  can_mb_idx=44  can_extended_id=on  can_is_remote=off  can_id=180128D0  show_adv_opts=off  can_fd_enable=off  can_enable_brs=off  can_fd_padding=0
      settings: SourceProductName=NXP Model-Based Design Toolbox for MPC57xx MCUs
  FCAN_Send_ID_0x180328D0 : mbd_mpc574x_ec_toolbox/Communication Blocks/CAN Blocks/FCAN_Send  Priority=2  can_instance=0  can_mode=Non-blocking  can_timeout_ms=0  can_mb_idx=44  can_extended_id=on  can_is_remote=off  can_id=180328D0  show_adv_opts=off  can_fd_enable=off  can_enable_brs=off  can_fd_padding=0
      settings: SourceProductName=NXP Model-Based Design Toolbox for MPC57xx MCUs
  FCAN_Send_ID_0x181128D0 : mbd_mpc574x_ec_toolbox/Communication Blocks/CAN Blocks/FCAN_Send  Priority=2  can_instance=0  can_mode=Non-blocking  can_timeout_ms=0  can_mb_idx=44  can_extended_id=on  can_is_remote=off  can_id=181128D0  show_adv_opts=off  can_fd_enable=off  can_enable_brs=off  can_fd_padding=0
      settings: SourceProductName=NXP Model-Based Design Toolbox for MPC57xx MCUs
  FCAN_Send_ID_0x181228D0 : mbd_mpc574x_ec_toolbox/Communication Blocks/CAN Blocks/FCAN_Send  Priority=2  can_instance=0  can_mode=Non-blocking  can_timeout_ms=0  can_mb_idx=44  can_extended_id=on  can_is_remote=off  can_id=181228D0  show_adv_opts=off  can_fd_enable=off  can_enable_brs=off  can_fd_padding=0
      settings: SourceProductName=NXP Model-Based Design Toolbox for MPC57xx MCUs
  FCAN_Send_ID_0x181328D0 : mbd_mpc574x_ec_toolbox/Communication Blocks/CAN Blocks/FCAN_Send  Priority=2  can_instance=1  can_mode=Non-blocking  can_timeout_ms=0  can_mb_idx=44  can_extended_id=on  can_is_remote=off  can_id=181328D0  show_adv_opts=off  can_fd_enable=off  can_enable_brs=off  can_fd_padding=0
      settings: SourceProductName=NXP Model-Based Design Toolbox for MPC57xx MCUs
  FCAN_Send_ID_0x181428D0 : mbd_mpc574x_ec_toolbox/Communication Blocks/CAN Blocks/FCAN_Send  Priority=2  can_instance=1  can_mode=Non-blocking  can_timeout_ms=0  can_mb_idx=44  can_extended_id=on  can_is_remote=off  can_id=181428D0  show_adv_opts=off  can_fd_enable=off  can_enable_brs=off  can_fd_padding=0
      settings: SourceProductName=NXP Model-Based Design Toolbox for MPC57xx MCUs
  VCU2MCU1_1 : canmsglib/CAN Pack  CANdbFile=D:\VCU\VCU_SL_ZhengZhou\ZT2\模型与接口\CAN_DBC\整车CANA_GBK.dbc  MsgList=VCU2ICUInfor1  MsgName=VCU2ICUInfor1  MsgIDType=Extended (29-bit identifier)  MsgIdentifier=402729168  MsgLength=8  SignalInfo=VCU_BattSOC_pct$16$8$1$2$1$0$1$0$0$100$#VCU_BattTempHi_b$32$1$1$2$1$0$1$0$0$1$#VCU_BrakeFlt_b$39$1$1$2$1$0$1$0$0$1$#VCU_CoolFanWrkIdc_b$44$1$1$2$1$0$1$0$0$1$#VCU_CoolSysFanPWM$56$8$1$2$1$0$1$0$0$100$#VCU_CoolSysFltIdc_b$43$1$1$2$1$0$1$0$0$1$#VCU_EmrPumpSt_enum$5$2$1$2$1$0$1$0$0$3$#VCU_FltSt_enum$6$1$1$2$1$0$1$0$0$1$#VCU_GearSt_enum$24$8$1$2$1$0$1$0$0$5$#VCU_HeadLight_b$46$1$1$2$1$0$1$0$0$1$#VCU_HydSysFlt_b$33$1$1$2$1$0$1$0$0$1$#VCU_LShift_b$3$1$1$2$1$0$1$0$0$1$#VCU_MCUTempHiFlt_b$35$1$1$2$1$0$1$0$0$1$#VCU_MtTempHiFlt_b$36$1$1$2$1$0$1$0$0$1$#VCU_Pst_b$0$1$1$2$1$0$1$0$0$1$#VCU_RShift_b$2$1$1$2$1$0$1$0$0$1$#VCU_RearLight_b$45$1$1$2$1$0$1$0$0$1$#VCU_SOCLoFlt_b$1$1$1$2$1$0$1$0$0$1$#VCU_SysWorkStCode_num$48$8$1$2$1$0$1$0$0$255$#VCU_TopWrkSt_b$38$1$1$2$1$0$1$0$0$1$#VCU_VehACharge_b$34$1$1$2$1$0$1$0$0$1$#VCU_VehDCharge_b$37$1$1$2$1$0$1$0$0$1$#VCU_VehSpd_kmh$8$8$1$2$1$0$1$0$0$255$#VCU_WatPumpOpenSt_b$47$1$1$2$1$0$1$0$0$1$#VCU_WrkSt_enum$7$1$1$2$1$0$1$0$0$1$#  NSignals=25  StartBits=str2num('[int32(16);int32(32);int32(39);int32(44);int32(56);int32(43);int32(5);int32(6);int32(24);int32(46);int32(33);int32(3);int32(35);int32(36);int32(0);int32(2);int32(45);int32(1);int32(48);int32(38);int32(34);int32(37);int32(8);int32(47);int32(7)]')  SignalSizes=str2num('[int32(8);int32(1);int32(1);int32(1);int32(8);int32(1);int32(2);int32(1);int32(8);int32(1);int32(1);int32(1);int32(1);int32(1);int32(1);int32(1);int32(1);int32(1);int32(8);int32(1);int32(1);int32(1);int32(8);int32(1);int32(1)]')  ByteOrders=str2num('[int32(1);int32(1);int32(1);int32(1);int32(1);int32(1);int32(1);int32(1);int32(1);int32(1);int32(1);int32(1);int32(1);int32(1);int32(1);int32(1);int32(1);int32(1);int32(1);int32(1);int32(1);int32(1);int32(1);int32(1);int32(1)]')  DataTypes=str2num('[int32(2);int32(2);int32(2);int32(2);int32(2);int32(2);int32(2);int32(2);int32(2);int32(2);int32(2);int32(2);int32(2);int32(2);int32(2);int32(2);int32(2);int32(2);int32(2);int32(2);int32(2);int32(2);int32(2);int32(2);int32(2)]')  MultiplexTypes=str2num('[int32(1);int32(1);int32(1);int32(1);int32(1);int32(1);int32(1);int32(1);int32(1);int32(1);int32(1);int32(1);int32(1);int32(1);int32(1);int32(1);int32(1);int32(1);int32(1);int32(1);int32(1);int32(1);int32(1);int32(1);int32(1)]')  MultiplexValues=str2num('[double(0);double(0);double(0);double(0);double(0);double(0);double(0);double(0);double(0);double(0);double(0);double(0);double(0);double(0);double(0);double(0);double(0);double(0);double(0);double(0);double(0);double(0);double(0);double(0);double(0)]')  Factors=str2num('[double(1);double(1);double(1);double(1);double(1);double(1);double(1);double(1);double(1);double(1);double(1);double(1);double(1);double(1);double(1);double(1);double(1);double(1);double(1);double(1);double(1);double(1);double(1);double(1);double(1)]')  Offsets=str2num('[double(0);double(0);double(0);double(0);double(0);double(0);double(0);double(0);double(0);double(0);double(0);double(0);double(0);double(0);double(0);double(0);double(0);double(0);double(0);double(0);double(0);double(0);double(0);double(0);double(0)]')  Minimums=str2num('[double(0);double(0);double(0);double(0);double(0);double(0);double(0);double(0);double(0);double(0);double(0);double(0);double(0);double(0);double(0);double(0);double(0);double(0);double(0);double(0);double(0);double(0);double(0);double(0);double(0)]')  Maximums=str2num('[double(100);double(1);double(1);double(1);double(100);double(1);double(3);double(1);double(5);double(1);double(1);double(1);double(1);double(1);double(1);double(1);double(1);double(1);double(255);double(1);double(1);double(1);double(255);double(1);double(1)]')  Remote=off  ApplyMinMax=off  BusOutput=on
      settings: SourceProductName=Simulink Real-Time  SourceProductBaseCode=XP  DataFormat=CANdb specified signals
  VCU2MCU1_3 : canmsglib/CAN Pack  CANdbFile=D:\VCU\VCU_SL_ZhengZhou\ZT2\模型与接口\CAN_DBC\整车CANA_GBK.dbc  MsgList=VCU2ICUInfor3  MsgName=VCU2ICUInfor3  MsgIDType=Extended (29-bit identifier)  MsgIdentifier=402860240  MsgLength=8  SignalInfo=VCU_BattBusVolt_V$48$16$1$2$1$0$1.000000e-01$0$0$6.553500e+03$#VCU_EVFltCode1_num$24$8$1$2$1$0$1$0$0$255$#VCU_EVFltCode2_num$32$8$1$2$1$0$1$0$0$255$#VCU_EVFltLvlMax_num$40$8$1$2$1$0$1$0$0$3$#VCU_HistFltCode1_num$0$8$1$2$1$0$1$0$0$255$#VCU_HistFltCode2_num$8$8$1$2$1$0$1$0$0$255$#VCU_HistFltCode3_num$16$8$1$2$1$0$1$0$0$255$#  NSignals=7  StartBits=str2num('[int32(48);int32(24);int32(32);int32(40);int32(0);int32(8);int32(16)]')  SignalSizes=str2num('[int32(16);int32(8);int32(8);int32(8);int32(8);int32(8);int32(8)]')  ByteOrders=str2num('[int32(1);int32(1);int32(1);int32(1);int32(1);int32(1);int32(1)]')  DataTypes=str2num('[int32(2);int32(2);int32(2);int32(2);int32(2);int32(2);int32(2)]')  MultiplexTypes=str2num('[int32(1);int32(1);int32(1);int32(1);int32(1);int32(1);int32(1)]')  MultiplexValues=str2num('[double(0);double(0);double(0);double(0);double(0);double(0);double(0)]')  Factors=str2num('[double(1.000000e-01);double(1);double(1);double(1);double(1);double(1);double(1)]')  Offsets=str2num('[double(0);double(0);double(0);double(0);double(0);double(0);double(0)]')  Minimums=str2num('[double(0);double(0);double(0);double(0);double(0);double(0);double(0)]')  Maximums=str2num('[double(6.553500e+03);double(255);double(255);double(3);double(255);double(255);double(255)]')  Remote=off  ApplyMinMax=off  BusOutput=on
      settings: SourceProductName=Simulink Real-Time  SourceProductBaseCode=XP  DataFormat=CANdb specified signals
  VCU2MCU1_4 : canmsglib/CAN Pack  CANdbFile=D:\VCU\VCU_SL_ZhengZhou\ZT2\模型与接口\CAN_DBC\整车CANA_GBK.dbc  MsgList=VCU2ICUInfor4  MsgName=VCU2ICUInfor4  MsgIDType=Extended (29-bit identifier)  MsgIdentifier=403777744  MsgLength=8  SignalInfo=VCU_BattTempMax_deg$48$8$1$1$1$0$1$-40$-40$215$#VCU_BattTempMin_deg$40$8$1$1$1$0$1$-40$-40$215$#VCU_CoolWaterTemp_deg$16$8$1$1$1$0$1$-40$-40$215$#VCU_DrvMtCtlUnitTemp_deg$32$8$1$1$1$0$1$-40$-40$215$#VCU_DrvMtTemp_deg$24$8$1$1$1$0$1$-40$-40$215$#VCU_OilMtCtlUnitTemp_deg$8$8$1$1$1$0$1$-40$-40$215$#VCU_OilMtTemp_deg$0$8$1$1$1$0$1$-40$-40$215$#VCU_RemindInfor_num$56$8$1$2$1$0$1$0$-Inf$Inf$#  NSignals=8  StartBits=str2num('[int32(48);int32(40);int32(16);int32(32);int32(24);int32(8);int32(0);int32(56)]')  SignalSizes=str2num('[int32(8);int32(8);int32(8);int32(8);int32(8);int32(8);int32(8);int32(8)]')  ByteOrders=str2num('[int32(1);int32(1);int32(1);int32(1);int32(1);int32(1);int32(1);int32(1)]')  DataTypes=str2num('[int32(1);int32(1);int32(1);int32(1);int32(1);int32(1);int32(1);int32(2)]')  MultiplexTypes=str2num('[int32(1);int32(1);int32(1);int32(1);int32(1);int32(1);int32(1);int32(1)]')  MultiplexValues=str2num('[double(0);double(0);double(0);double(0);double(0);double(0);double(0);double(0)]')  Factors=str2num('[double(1);double(1);double(1);double(1);double(1);double(1);double(1);double(1)]')  Offsets=str2num('[double(-40);double(-40);double(-40);double(-40);double(-40);double(-40);double(-40);double(0)]')  Minimums=str2num('[double(-40);double(-40);double(-40);double(-40);double(-40);double(-40);double(-40);double(-Inf)]')  Maximums=str2num('[double(215);double(215);double(215);double(215);double(215);double(215);double(215);double(Inf)]')  Remote=off  ApplyMinMax=off  BusOutput=on
      settings: SourceProductName=Simulink Real-Time  SourceProductBaseCode=XP  DataFormat=CANdb specified signals
  VCU2MCU1_5 : canmsglib/CAN Pack  CANdbFile=D:\VCU\VCU_SL_ZhengZhou\ZT2\模型与接口\CAN_DBC\整车CANA_GBK.dbc  MsgList=VCU2ICUInfor5  MsgName=VCU2ICUInfor5  MsgIDType=Extended (29-bit identifier)  MsgIdentifier=403843280  MsgLength=8  SignalInfo=VCU_DrvMCUBusCurr_A$48$16$1$1$1$0$1$-1000$-1000$35535$#VCU_DrvMCUBusVolt_V$32$16$1$2$1$0$1$0$0$65535$#VCU_DrvMtSpd_rpm$0$16$1$1$1$0$1$-30000$-30000$35535$#VCU_DrvMtTrq_Nm$16$16$1$2$1$0$1$0$0$65535$#  NSignals=4  StartBits=str2num('[int32(48);int32(32);int32(0);int32(16)]')  SignalSizes=str2num('[int32(16);int32(16);int32(16);int32(16)]')  ByteOrders=str2num('[int32(1);int32(1);int32(1);int32(1)]')  DataTypes=str2num('[int32(1);int32(2);int32(1);int32(2)]')  MultiplexTypes=str2num('[int32(1);int32(1);int32(1);int32(1)]')  MultiplexValues=str2num('[double(0);double(0);double(0);double(0)]')  Factors=str2num('[double(1);double(1);double(1);double(1)]')  Offsets=str2num('[double(-1000);double(0);double(-30000);double(0)]')  Minimums=str2num('[double(-1000);double(0);double(-30000);double(0)]')  Maximums=str2num('[double(35535);double(65535);double(35535);double(65535)]')  Remote=off  ApplyMinMax=off  BusOutput=on
      settings: SourceProductName=Simulink Real-Time  SourceProductBaseCode=XP  DataFormat=CANdb specified signals
  VCU2MCU1_6 : canmsglib/CAN Pack  CANdbFile=D:\VCU\VCU_SL_ZhengZhou\ZT2\模型与接口\CAN_DBC\整车CANA_GBK.dbc  MsgList=VCU2ICUInfor6  MsgName=VCU2ICUInfor6  MsgIDType=Extended (29-bit identifier)  MsgIdentifier=403908816  MsgLength=8  SignalInfo=VCU_OilMCUBusCurr_A$48$16$1$1$1$0$1$-1000$-1000$35535$#VCU_OilMCUBusVolt_V$32$16$1$2$1$0$1$0$0$65535$#VCU_OilMtSpd_rpm$0$16$1$2$1$0$1$0$0$65535$#VCU_OilMtTrq_Nm$16$16$1$2$1$0$1$0$0$65535$#  NSignals=4  StartBits=str2num('[int32(48);int32(32);int32(0);int32(16)]')  SignalSizes=str2num('[int32(16);int32(16);int32(16);int32(16)]')  ByteOrders=str2num('[int32(1);int32(1);int32(1);int32(1)]')  DataTypes=str2num('[int32(1);int32(2);int32(2);int32(2)]')  MultiplexTypes=str2num('[int32(1);int32(1);int32(1);int32(1)]')  MultiplexValues=str2num('[double(0);double(0);double(0);double(0)]')  Factors=str2num('[double(1);double(1);double(1);double(1)]')  Offsets=str2num('[double(-1000);double(0);double(0);double(0)]')  Minimums=str2num('[double(-1000);double(0);double(0);double(0)]')  Maximums=str2num('[double(35535);double(65535);double(65535);double(65535)]')  Remote=off  ApplyMinMax=off  BusOutput=on
      settings: SourceProductName=Simulink Real-Time  SourceProductBaseCode=XP  DataFormat=CANdb specified signals
  VCU2MCU1_7 : canmsglib/CAN Pack  CANdbFile=D:\VCU\VCU_SL_ZhengZhou\ZT2\模型与接口\CAN_DBC\整车CANA_GBK.dbc  MsgList=VCU2ICUInfor7  MsgName=VCU2ICUInfor7  MsgIDType=Extended (29-bit identifier)  MsgIdentifier=403974352  MsgLength=8  SignalInfo=VCU_DisChargePwr_kw$0$16$1$2$1$0$1.000000e-01$0$0$10000$#VCU_RangeRemain_km$48$16$1$2$1$0$1$0$0$65535$#VCU_RegenPwr_kw$16$16$1$2$1$0$1.000000e-01$0$0$10000$#VCU_RunAllMile_km$32$16$1$2$1$0$1$0$0$65535$#  NSignals=4  StartBits=str2num('[int32(0);int32(48);int32(16);int32(32)]')  SignalSizes=str2num('[int32(16);int32(16);int32(16);int32(16)]')  ByteOrders=str2num('[int32(1);int32(1);int32(1);int32(1)]')  DataTypes=str2num('[int32(2);int32(2);int32(2);int32(2)]')  MultiplexTypes=str2num('[int32(1);int32(1);int32(1);int32(1)]')  MultiplexValues=str2num('[double(0);double(0);double(0);double(0)]')  Factors=str2num('[double(1.000000e-01);double(1);double(1.000000e-01);double(1)]')  Offsets=str2num('[double(0);double(0);double(0);double(0)]')  Minimums=str2num('[double(0);double(0);double(0);double(0)]')  Maximums=str2num('[double(10000);double(65535);double(10000);double(65535)]')  Remote=off  ApplyMinMax=off  BusOutput=on
      settings: SourceProductName=Simulink Real-Time  SourceProductBaseCode=XP  DataFormat=CANdb specified signals
  wires:
  VCU2MCU1_1/1 -> Bus Selector/1
  "ICU_OUT "/1 -> Bus Selector1/1
  Bus Selector/1 -> FCAN_Send_ID_0x180128D0/1  "<Data>"
  Bus Selector/2 -> FCAN_Send_ID_0x180128D0/2  "<Length>"
  VCU2MCU1_3/1 -> Bus Selector3/1
  Bus Selector3/1 -> FCAN_Send_ID_0x180328D0/1  "<Data>"
  Bus Selector3/2 -> FCAN_Send_ID_0x180328D0/2  "<Length>"
  Bus Selector4/2 -> FCAN_Send_ID_0x181128D0/2  "<Length>"
  Bus Selector4/1 -> FCAN_Send_ID_0x181128D0/1  "<Data>"
  VCU2MCU1_4/1 -> Bus Selector4/1
  VCU2MCU1_5/1 -> Bus Selector5/1
  Bus Selector5/1 -> FCAN_Send_ID_0x181228D0/1  "<Data>"
  Bus Selector5/2 -> FCAN_Send_ID_0x181228D0/2  "<Length>"
  Bus Selector6/2 -> FCAN_Send_ID_0x181328D0/2  "<Length>"
  Bus Selector6/1 -> FCAN_Send_ID_0x181328D0/1  "<Data>"
  VCU2MCU1_6/1 -> Bus Selector6/1
  VCU2MCU1_7/1 -> Bus Selector7/1
  Bus Selector7/1 -> FCAN_Send_ID_0x181428D0/1  "<Data>"
  Bus Selector7/2 -> FCAN_Send_ID_0x181428D0/2  "<Length>"
